simulink model "LWDF_butter3"  (R2016a)
settings: Solver=ode45  StartTime=0.0  StopTime=10.0  RelTol=1e-3
undefined symbols (not defined in the file or in its folder): g1, g2, g3
settings Model: Creator=anastasiialozanova  LastModifiedBy=thib
settings DataIOCC: LimitDataPoints=on  SaveFormat=Array
settings DebuggingCC: SolverPrmCheckMsg=warning
settings HardwareCC: ProdBitPerPointer=32  ProdLargestAtomicFloat=None  ProdIntDivRoundTo=Undefined  ProdEndianess=Unspecified  ProdWordSize=32  ProdHWDeviceType=32-bit Generic
settings ModelReferenceCC: PropagateSignalLabelsOutOfModel=off
settings ConfigComp: CovModelRefEnable=Off  CovSFcnEnable=off

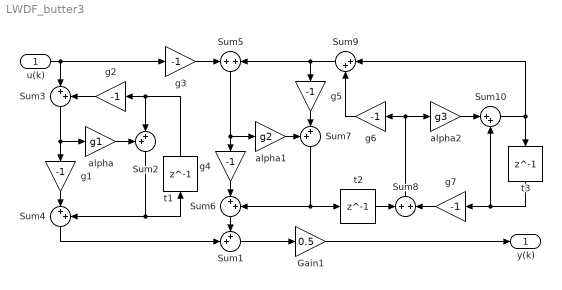
== system LWDF_butter3 ==
  u(k) : Inport
  Gain1 : Gain  Gain=0.5
  Sum1 : Sum  Inputs=++|
  Sum{3..4,6,9..10} (5 alike) : Sum  Inputs=|++
  Sum2 : Sum  Inputs=++|
  Sum5 : Sum  Inputs=+|+
  Sum7 : Sum  Inputs=++|
  Sum8 : Sum  Inputs=+|+
  alpha : Gain  Gain=g1
  alpha1 : Gain  Gain=g2
  alpha2 : Gain  Gain=g3
  g{1..7} (7 alike) : Gain  Gain=-1
  t1 : Delay  DelayLength=1  InitialCondition=0
  t2 : Delay  DelayLength=1  InitialCondition=0
  t3 : Delay  DelayLength=1  InitialCondition=0
  y(k) : Outport
  wires:
  Sum2/1 -> Sum4/2, t1/1
  Sum7/1 -> t2/1, Sum6/2
  Sum10/1 -> Sum9/1, t3/1
  Sum4/1 -> Sum1/2
  Sum1/1 -> Gain1/1
  Sum6/1 -> Sum1/1
  alpha/1 -> Sum2/1
  Sum3/1 -> g1/1, alpha/1
  g1/1 -> Sum4/1
  t1/1 -> Sum2/2, g2/1
  g2/1 -> Sum3/2
  g5/1 -> Sum7/2
  g3/1 -> Sum5/1
  alpha1/1 -> Sum7/1
  Sum5/1 -> alpha1/1, g4/1
  g4/1 -> Sum6/1
  u(k)/1 -> g3/1, Sum3/1
  Sum9/1 -> g5/1, Sum5/2
  Sum8/1 -> alpha2/1, g6/1
  g6/1 -> Sum9/2
  t2/1 -> Sum8/1
  t3/1 -> Sum10/2, g7/1
  g7/1 -> Sum8/2
  Gain1/1 -> y(k)/1
  alpha2/1 -> Sum10/1
